simulink model "test_c2000"  (R2025a)
settings: Solver=FixedStepAuto  StartTime=0.0  StopTime=200  RelTol=1e-3  EnableMultiTasking=on
undefined symbols (not defined in the file or in its folder): bit
libraries: c2802xlib x1
settings Model: Creator=mafur  LastModifiedBy=mafur
settings OptimizationCC: DefaultParameterBehavior=Inlined  DefaultUnderspecifiedDataType=single  EnhancedBackFolding=on  PassReuseOutputArgsAs=Individual arguments  ZeroExternalMemoryAtStartup=off  MaxStackSize=64  OptimizeBlockOrder=speed  DifferentSizesBufferReuse=on  OptimizationCustomize=off  EfficientTunableParamExpr=on
settings DebuggingCC: ParameterTunabilityLossMsg=error
settings HardwareCC: ProdBitPerChar=16.0  ProdBitPerInt=16.0  ProdBitPerPointer=32.0  ProdBitPerSizeT=32.0  ProdBitPerPtrDiffT=32.0  ProdLargestAtomicInteger=Integer  ProdLargestAtomicFloat=None  ProdWordSize=16.0  ProdHWDeviceType=Texas Instruments->C2000  HardwareBoardFeatureSet=SoCBlockset
settings SFSimCC: MATLABDynamicMemAlloc=off
settings RTWCC: SystemTargetFile=ert.tlc  HardwareBoard=TI Delfino F28379D LaunchPad  TemplateMakefile=ert_default_tmf  RTWUseSimCustomCode=on  Toolchain=Texas Instruments Code Composer Studio (C2000)  Description=Embedded Coder
settings CodeAppCC: ForceParamTrailComments=on  IgnoreCustomStorageClasses=off  OperatorAnnotations=on  SimulinkDataObjDesc=on  SFDataObjDesc=on  InsertBlockDesc=on
settings ERTTargetCC: ExtModeTransport=4.0  ExtModeStaticAllocSize=10000.0  SuppressErrorStatus=on

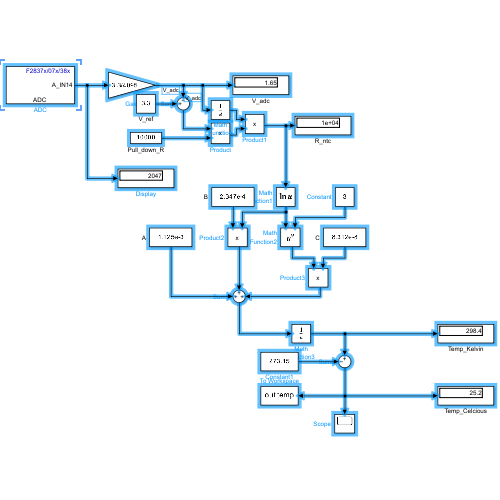
[thumbnail: Simulink's stored preview of the top-level diagram]
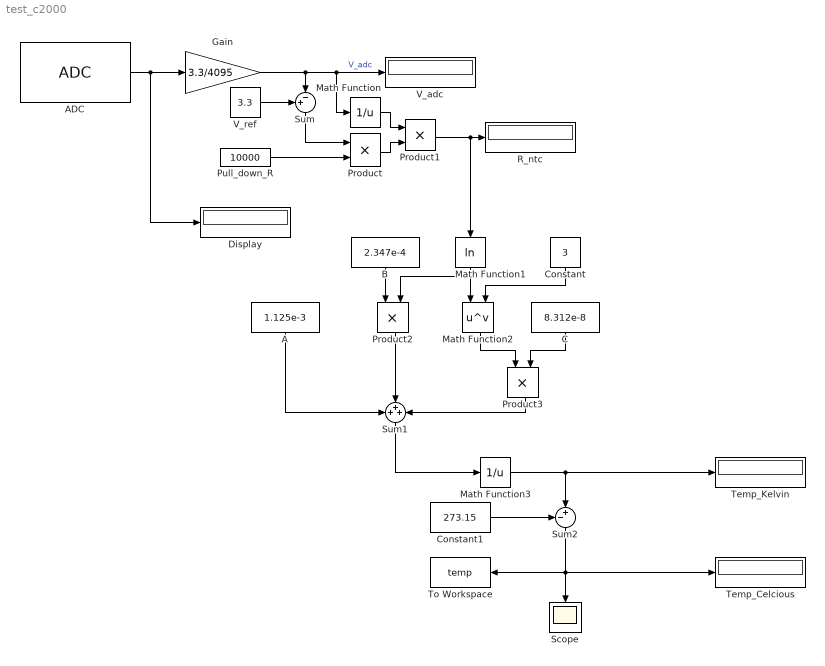
== system test_c2000 ==
  A : Constant  Value=1.125e-3
  ADC : c2802xlib/ADC  blkParamProc=C2000_Type4  ADCModule=A  samplingMode=Single sample mode  ADCResolution=12-bit (Single-ended input)  ADC29xResolution=12-bit  ADCMode=Single-ended input  useSOC1=SOC0  useSOC2=SOC0_SOC1  SOCAcquisitionWindow=15  SOCTriggerSource=Software  SOCInterruptTrigger=No ADCINT  Ts=0.1  dType=int32  postInterrupt=off  interruptSel=ADCINT1  ADCINTContinuous=on  endma=off  chdma=1  conv1=ADCINA0  conv2=ADCINA0 and ADCINB0  conv1_Type4=ADCIN14  conv2_Type4=ADCIN0 and ADCIN1
      settings: LibrarySourceBlock=c2837xDlib/ADC
  B : Constant  Value=2.347e-4
  C : Constant  Value=8.312e-8
  Constant : Constant  Value=3
  Constant1 : Constant  Value=273.15
  Display : Display
  Gain : Gain  Gain=3.3/4095
  Math Function : Math  Operator=reciprocal
  Math Function1 : Math  Operator=log
  Math Function2 : Math  Operator=pow
  Math Function3 : Math  Operator=reciprocal
  Product{,1..3} (4 alike) : Product
  Pull_down_R : Constant  Value=10000
  R_ntc : Display
  Scope : Scope
      settings: ActiveDisplayYMinimum=12.472118117855352  ActiveDisplayYMaximum=14.326535623482876
  Sum : Sum  Inputs=+-|
  Sum1 : Sum  Inputs=+++
  Sum2 : Sum  Inputs=-+|
  Temp_Celcious : Display
  Temp_Kelvin : Display
  To Workspace : ToWorkspace  VariableName=temp  SaveFormat=Timeseries  SampleTime=-1
  V_adc : Display
  V_ref : Constant  Value=3.3
  wires:
  Math Function1/1 -> Math Function2/1, Product2/2
  Math Function3/1 -> Sum2/2, Temp_Kelvin/1
  ADC/1 -> Display/1, Gain/1
  Gain/1 -> Sum/2, Math Function/1, V_adc/1  "V_adc"
  V_ref/1 -> Sum/1
  Sum/1 -> Product/1
  Pull_down_R/1 -> Product/2
  Product/1 -> Product1/2
  Math Function/1 -> Product1/1
  Product1/1 -> Math Function1/1, R_ntc/1
  Constant/1 -> Math Function2/2
  B/1 -> Product2/1
  A/1 -> Sum1/1
  Product2/1 -> Sum1/2
  Product3/1 -> Sum1/3
  Math Function2/1 -> Product3/1
  C/1 -> Product3/2
  Sum1/1 -> Math Function3/1
  Constant1/1 -> Sum2/1
  Sum2/1 -> Scope/1, To Workspace/1, Temp_Celcious/1
